simulink model "v2012_DynStab"  (Simulink 7.6)
settings: Solver=ode45  StartTime=0.0  StopTime=10.0  RelTol=1e-3
libraries: fm_lib x1
(part 4 of 4)

== system v2012_DynStab/AVR1 ==
  note: Automatic Voltage Regulator
  Constant : Constant
  Out1 : Outport
  wires:
  Constant/1 -> Out1/1

== system v2012_DynStab/AVR10 ==
  note: Automatic Voltage Regulator
  Constant : Constant
  Out1 : Outport
  wires:
  Constant/1 -> Out1/1

== system v2012_DynStab/AVR11 ==
  note: Automatic Voltage Regulator
  Constant : Constant
  Out1 : Outport
  wires:
  Constant/1 -> Out1/1

== system v2012_DynStab/AVR12 ==
  note: Automatic Voltage Regulator
  Constant : Constant
  Out1 : Outport
  wires:
  Constant/1 -> Out1/1

== system v2012_DynStab/AVR13 ==
  note: Automatic Voltage Regulator
  Constant : Constant
  Out1 : Outport
  wires:
  Constant/1 -> Out1/1

== system v2012_DynStab/AVR2 ==
  note: Automatic Voltage Regulator
  Constant : Constant
  Out1 : Outport
  wires:
  Constant/1 -> Out1/1

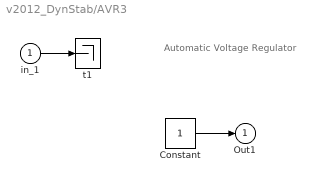
== system v2012_DynStab/AVR3 ==
  note: Automatic Voltage Regulator
  in_1 : Inport
  Constant : Constant
  t1 : Terminator
  Out1 : Outport
  wires:
  Constant/1 -> Out1/1
  in_1/1 -> t1/1

== system v2012_DynStab/AVR4 ==
  note: Automatic Voltage Regulator
  Constant : Constant
  Out1 : Outport
  wires:
  Constant/1 -> Out1/1

== system v2012_DynStab/AVR5 ==
  note: Automatic Voltage Regulator
  Constant : Constant
  Out1 : Outport
  wires:
  Constant/1 -> Out1/1

== system v2012_DynStab/AVR6 ==
  note: Automatic Voltage Regulator
  Constant : Constant
  Out1 : Outport
  wires:
  Constant/1 -> Out1/1

== system v2012_DynStab/AVR7 ==
  note: Automatic Voltage Regulator
  Constant : Constant
  Out1 : Outport
  wires:
  Constant/1 -> Out1/1

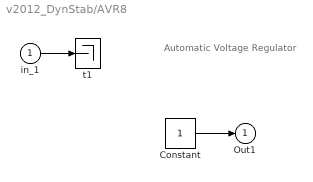
== system v2012_DynStab/AVR8 ==
  note: Automatic Voltage Regulator
  in_1 : Inport
  Constant : Constant
  t1 : Terminator
  Out1 : Outport
  wires:
  Constant/1 -> Out1/1
  in_1/1 -> t1/1

== system v2012_DynStab/Pss ==
  note: Power System Stabilizer
  Constant : Constant
  Out1 : Outport
  wires:
  Constant/1 -> Out1/1

== system v2012_DynStab/Pss1 ==
  note: Power System Stabilizer
  Constant : Constant
  Out1 : Outport
  wires:
  Constant/1 -> Out1/1

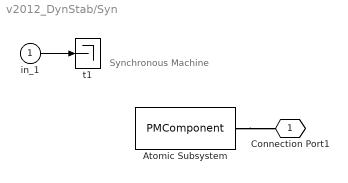
== system v2012_DynStab/Syn ==
  note: Synchronous Machine
  in_1 : Inport
  Atomic Subsystem : PMComponent  PhysicalDomain=psatdomain  LeftPortType=p1  RightPortType=p1  RConnTagsString=__newr0
  t1 : Terminator
  Connection Port1 : PMIOPort  Tag=PMCPort  Port=1  Side=Right
  wires:
  in_1/1 -> t1/1
  connections:
  Atomic Subsystem/RConn1 -- Connection Port1/RConn1

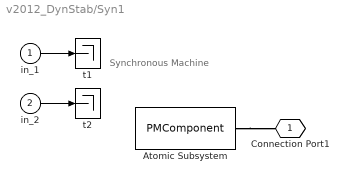
== system v2012_DynStab/Syn1 ==
  note: Synchronous Machine
  in_1 : Inport
  in_2 : Inport  Port=2
  Atomic Subsystem : PMComponent  PhysicalDomain=psatdomain  LeftPortType=p1  RightPortType=p1  RConnTagsString=__newr0
  t1 : Terminator
  t2 : Terminator
  Connection Port1 : PMIOPort  Tag=PMCPort  Port=1  Side=Right
  wires:
  in_1/1 -> t1/1
  in_2/1 -> t2/1
  connections:
  Atomic Subsystem/RConn1 -- Connection Port1/RConn1

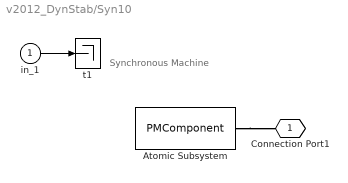
== system v2012_DynStab/Syn10 ==
  note: Synchronous Machine
  in_1 : Inport
  Atomic Subsystem : PMComponent  PhysicalDomain=psatdomain  LeftPortType=p1  RightPortType=p1  RConnTagsString=__newr0
  t1 : Terminator
  Connection Port1 : PMIOPort  Tag=PMCPort  Port=1  Side=Right
  wires:
  in_1/1 -> t1/1
  connections:
  Atomic Subsystem/RConn1 -- Connection Port1/RConn1

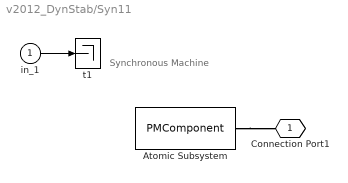
== system v2012_DynStab/Syn11 ==
  note: Synchronous Machine
  in_1 : Inport
  Atomic Subsystem : PMComponent  PhysicalDomain=psatdomain  LeftPortType=p1  RightPortType=p1  RConnTagsString=__newr0
  t1 : Terminator
  Connection Port1 : PMIOPort  Tag=PMCPort  Port=1  Side=Right
  wires:
  in_1/1 -> t1/1
  connections:
  Atomic Subsystem/RConn1 -- Connection Port1/RConn1

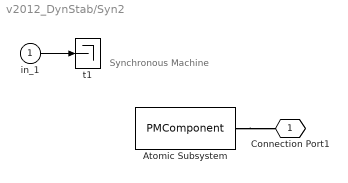
== system v2012_DynStab/Syn2 ==
  note: Synchronous Machine
  in_1 : Inport
  Atomic Subsystem : PMComponent  PhysicalDomain=psatdomain  LeftPortType=p1  RightPortType=p1  RConnTagsString=__newr0
  t1 : Terminator
  Connection Port1 : PMIOPort  Tag=PMCPort  Port=1  Side=Right
  wires:
  in_1/1 -> t1/1
  connections:
  Atomic Subsystem/RConn1 -- Connection Port1/RConn1

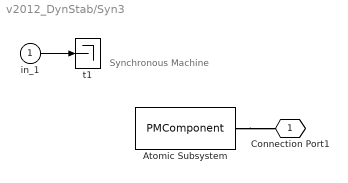
== system v2012_DynStab/Syn3 ==
  note: Synchronous Machine
  in_1 : Inport
  Atomic Subsystem : PMComponent  PhysicalDomain=psatdomain  LeftPortType=p1  RightPortType=p1  RConnTagsString=__newr0
  t1 : Terminator
  Connection Port1 : PMIOPort  Tag=PMCPort  Port=1  Side=Right
  wires:
  in_1/1 -> t1/1
  connections:
  Atomic Subsystem/RConn1 -- Connection Port1/RConn1

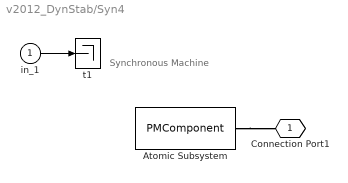
== system v2012_DynStab/Syn4 ==
  note: Synchronous Machine
  in_1 : Inport
  Atomic Subsystem : PMComponent  PhysicalDomain=psatdomain  LeftPortType=p1  RightPortType=p1  RConnTagsString=__newr0
  t1 : Terminator
  Connection Port1 : PMIOPort  Tag=PMCPort  Port=1  Side=Right
  wires:
  in_1/1 -> t1/1
  connections:
  Atomic Subsystem/RConn1 -- Connection Port1/RConn1

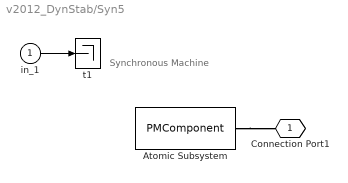
== system v2012_DynStab/Syn5 ==
  note: Synchronous Machine
  in_1 : Inport
  Atomic Subsystem : PMComponent  PhysicalDomain=psatdomain  LeftPortType=p1  RightPortType=p1  RConnTagsString=__newr0
  t1 : Terminator
  Connection Port1 : PMIOPort  Tag=PMCPort  Port=1  Side=Right
  wires:
  in_1/1 -> t1/1
  connections:
  Atomic Subsystem/RConn1 -- Connection Port1/RConn1

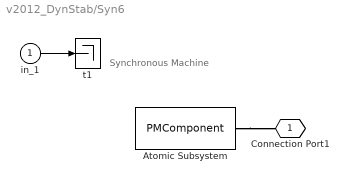
== system v2012_DynStab/Syn6 ==
  note: Synchronous Machine
  in_1 : Inport
  Atomic Subsystem : PMComponent  PhysicalDomain=psatdomain  LeftPortType=p1  RightPortType=p1  RConnTagsString=__newr0
  t1 : Terminator
  Connection Port1 : PMIOPort  Tag=PMCPort  Port=1  Side=Right
  wires:
  in_1/1 -> t1/1
  connections:
  Atomic Subsystem/RConn1 -- Connection Port1/RConn1

== system v2012_DynStab/Syn7 ==
  note: Synchronous Machine
  in_1 : Inport
  Atomic Subsystem : PMComponent  PhysicalDomain=psatdomain  LeftPortType=p1  RightPortType=p1  RConnTagsString=__newr0
  t1 : Terminator
  Connection Port1 : PMIOPort  Tag=PMCPort  Port=1  Side=Right
  wires:
  in_1/1 -> t1/1
  connections:
  Atomic Subsystem/RConn1 -- Connection Port1/RConn1

== system v2012_DynStab/Syn8 ==
  note: Synchronous Machine
  in_1 : Inport
  Atomic Subsystem : PMComponent  PhysicalDomain=psatdomain  LeftPortType=p1  RightPortType=p1  RConnTagsString=__newr0
  t1 : Terminator
  Connection Port1 : PMIOPort  Tag=PMCPort  Port=1  Side=Right
  wires:
  in_1/1 -> t1/1
  connections:
  Atomic Subsystem/RConn1 -- Connection Port1/RConn1

== system v2012_DynStab/Syn9 ==
  note: Synchronous Machine
  in_1 : Inport
  Atomic Subsystem : PMComponent  PhysicalDomain=psatdomain  LeftPortType=p1  RightPortType=p1  RConnTagsString=__newr0
  t1 : Terminator
  Connection Port1 : PMIOPort  Tag=PMCPort  Port=1  Side=Right
  wires:
  in_1/1 -> t1/1
  connections:
  Atomic Subsystem/RConn1 -- Connection Port1/RConn1

== system v2012_DynStab/Tg2 ==
  note: Turbine Governor
  Constant : Constant
  Out1 : Outport
  wires:
  Constant/1 -> Out1/1
